simulink model "Non_WindFarm"  (R2024a)
settings: Solver=ode45  StartTime=parSimulacio.ti  StopTime=200  MaxStep=parSimulacio.pas  RelTol=1e-6  AbsTol=1e-6  EnableMultiTasking=on
model workspace (MAT data in the model file):
  tt_vw : Simulink.Parameter (value not decoded)
values from neighbouring files (symbols this model uses):
  L = L'    [Lin_SignalGenerator.m]    (also in Non_ParameterInitialize.m; cal_QR.m = zeros(v, 1); parameters_windFarm2.m)
  nu = size(S, 1)    [Lin_SignalGenerator.m]    (also in Non_ParameterInitialize.m; parameters_windFarm2.m)
  S = zeros(v, v)    [cal_QR.m]
  w0 = [1 -0.00962521549583 0.0254779042049 -0.0160197396127 -0.0156056332727 0.0112137208272 0.0440607583301 -0.0193704893312 -0.0229464276306 -0.00247675309015 0.0285830611299]    [w0.mat]
undefined symbols (not defined in the file or in its folder): parControl, parConvertidor, parGenerador, parGrid, parMecanica, parSimulacio, windspeed
(part 26 of 40)

== system Non_WindFarm/FOM/Wind Farm/Wind Turbine Strings/String6/WT2/WFG/Maquina Sincrona ==
  note: Eq 4.22
  note: park transformation & Inverse
  note: theta_r
  note: Electrical angle=Mechnical angle *Pole Pairs
  note: Omega_r=Omega_m*P
  vsabc : Inport
  omega_m : Inport  Port=2
  theta_m : Inport  Port=3  PortDimensions=1
  Add : Sum  Inputs=+++
  Constant : Constant  Value=-rs/Lq
  Constant1 : Constant  Value=-rs/Ld
  Constant2 : Constant  Value=[1/Lq;0]
  Constant3 : Constant  Value=[1/Lq,0;0,1/Ld]
  Demux : Demux  Outputs=2
  Gain : Gain  Gain=-Ld/Lq
  Gain1 : Gain  Gain=Lq/Ld
  Gain2 : Gain  Gain=-lambda_m
  Gain3 : Gain  Gain=lambda_m
  Gain4 : Gain  Gain=Ld-Lq
  Gain5 : Gain  Gain=3/2*P
  Gain6 : Gain  Gain=P
  Gain7 : Gain  Gain=P
  Integrator : Integrator  InitialCondition=isqd0
  Matrix Concatenate : Concatenate  Mode=Multidimensional array  ConcatenateDimension=2
  Mux : Mux  Inputs=2
  Mux1 : Mux  Inputs=2
  Park : Subsystem
  Product{,2,4..5} (4 alike) : Product  Multiplication=Matrix(*)  RndMeth=Zero
  Product1 : Product  RndMeth=Zero
  Product3 : Product  RndMeth=Zero
  Sum : Sum  Inputs=|++
  isabc : Outport
  parell_m : Outport  Port=2
  wires:
  Constant/1 -> Mux/1
  Gain1/1 -> Mux/2
  Gain/1 -> Mux1/1
  Constant1/1 -> Mux1/2
  omega_m/1 -> Gain6/1
  Mux/1 -> Matrix Concatenate/1
  Mux1/1 -> Matrix Concatenate/2
  Matrix Concatenate/1 -> Product/1
  Product/1 -> Add/1
  Add/1 -> Integrator/1  "disqd"
  Integrator/1 -> Demux/1, Product5/2, Product/2  "isqd"
  Gain2/1 -> Product1/2
  Constant2/1 -> Product1/1
  Product1/1 -> Add/2
  Constant3/1 -> Product2/1
  Product2/1 -> Add/3
  Demux/1 -> Gain3/1, Product3/2
  Product3/1 -> Gain4/1
  Demux/2 -> Product3/1
  Gain3/1 -> Sum/1
  Gain4/1 -> Sum/2
  Sum/1 -> Gain5/1
  Gain5/1 -> parell_m/1
  Gain6/1 -> Gain1/1, Gain/1, Gain2/1
  theta_m/1 -> Gain7/1
  Product4/1 -> Product2/2
  Park/1(Tthetar) -> Product4/1
  Gain7/1 -> Park/1(theta_r)
  Park/2(nTthetar) -> Product5/1
  Product5/1 -> isabc/1
  vsabc/1 -> Product4/2

== system Non_WindFarm/FOM/Wind Farm/Wind Turbine Strings/String6/WT2/WFG/Mecanica nolineal i vent ==
  note: gearbox ration
  note: Gamma_t
  parell_m : Inport
  theta_a : Inport  Port=2
  vw : Inport  Port=3
  Gain1 : Gain  Gain=1/It
  Gain2 : Gain  Gain=nu
  Gain4 : Gain  Gain=nu
  Gain5 : Gain  Gain=nu
  Integrator : Integrator  InitialCondition=omegat0
  Integrator1 : Integrator
  Saturation : Saturate  UpperLimit=inf  LowerLimit=1e-6
  Sum : Sum  Inputs=++|
  Transfer Fcn : TransferFcn  Denominator=[taupitch 1]
  Turbina : Subsystem  mask{rho=1.225, R=R, cs=[0.5 116 0.4 0 0 5 21 0.08 0.035]}
      mask prompts: rho "Densitat de l'aire (Kg/m^3)"; R "Radi (R)"; cs "Constants [c1 c2 .. c9]"
      mask init:
      | A=pi*R^2;
      | c1=cs(1);
      | c2=cs(2);
      | c3=cs(3);
      | c4=cs(4);
      | c5=cs(5);
      | c6=cs(6);
      | c7=cs(7);
      | c8=cs(8);
      | c9=cs(9);
  omega_m : Outport
  theta_m : Outport  Port=2
  Cp : Outport  Port=3
  theta_aleps : Outport  Port=4
  wires:
  Sum/1 -> Gain1/1
  Gain1/1 -> Integrator/1
  Integrator/1 -> Integrator1/1, Gain4/1, Saturation/1
  Turbina/1(parell_turbina) -> Sum/2
  Gain2/1 -> Sum/1
  parell_m/1 -> Gain2/1
  Integrator1/1 -> Gain5/1
  Gain4/1 -> omega_m/1
  Gain5/1 -> theta_m/1
  Saturation/1 -> Turbina/2(omega_aleps)
  Turbina/2(Cp) -> Cp/1
  Transfer Fcn/1 -> theta_aleps/1, Turbina/3(theta_aleps)  "theta_aleps"
  theta_a/1 -> Transfer Fcn/1
  vw/1 -> Turbina/1(velocitat_vent)

== system Non_WindFarm/FOM/Wind Farm/Wind Turbine Strings/String6/WT2/WFG/Park ==
  theta_r : Inport
  Constant4 : Constant  Value=2*pi/3
  Gain7 : Gain  Gain=2/3
  Matrix Concatenate1 : Concatenate  NumInputs=3  Mode=Multidimensional array  ConcatenateDimension=2
  Matrix Concatenate2 : Concatenate  Mode=Multidimensional array  ConcatenateDimension=2
  Mux2 : Mux  Inputs=2
  Mux3 : Mux  Inputs=2
  Mux4 : Mux  Inputs=2
  Mux5 : Mux  Inputs=3
  Mux6 : Mux  Inputs=3
  Sum1 : Sum  Inputs=|++
  Sum2 : Sum  Inputs=|+-
  Trigonometric Function : Trigonometry  Operator=cos
  Trigonometric Function1 : Trigonometry
  Trigonometric Function2 : Trigonometry  Operator=cos
  Trigonometric Function3 : Trigonometry
  Trigonometric Function4 : Trigonometry  Operator=cos
  Trigonometric Function5 : Trigonometry
  Tthetar : Outport
  nTthetar : Outport  Port=2
  wires:
  theta_r/1 -> Sum1/1, Sum2/1, Trigonometric Function/1, Trigonometric Function1/1
  Sum2/1 -> Trigonometric Function2/1, Trigonometric Function3/1
  Sum1/1 -> Trigonometric Function4/1, Trigonometric Function5/1
  Constant4/1 -> Sum2/2, Sum1/2
  Trigonometric Function/1 -> Mux2/1, Mux5/1
  Trigonometric Function1/1 -> Mux2/2, Mux6/1
  Trigonometric Function2/1 -> Mux3/1, Mux5/2
  Trigonometric Function3/1 -> Mux3/2, Mux6/2
  Trigonometric Function4/1 -> Mux4/1, Mux5/3
  Trigonometric Function5/1 -> Mux4/2, Mux6/3
  Mux2/1 -> Matrix Concatenate1/1
  Mux3/1 -> Matrix Concatenate1/2
  Mux4/1 -> Matrix Concatenate1/3
  Matrix Concatenate1/1 -> Gain7/1
  Mux5/1 -> Matrix Concatenate2/1
  Mux6/1 -> Matrix Concatenate2/2
  Gain7/1 -> Tthetar/1
  Matrix Concatenate2/1 -> nTthetar/1

== system Non_WindFarm/FOM/Wind Farm/Wind Turbine Strings/String6/WT3/Transformer-complex/homopolar sequence ==
  note: Vc_cable_abc_bar
  note: Vc_cable_qd_bar
  note: WE
  note: Vc_filter_abc_bar
  note: Vc_filter_qd_bar
  Vc_cable_qd : Inport
  Vc_filter_qd : Inport  Port=2
  Clock : Clock
  Park : Subsystem
  Product{3..5,7} (4 alike) : Product  Multiplication=Matrix(*)  RndMeth=Zero
  homopolar sequence 1 : Subsystem
  homopolar sequence 2 : Subsystem
  we : Gain  Gain=100*pi
  Vc_cable_bar : Outport
  Vc_filter_bar : Outport  Port=2
  wires:
  Park/2(nTthetar) -> Product3/1, Product4/1
  Park/1(Tthetar) -> Product5/1, Product7/1
  Product4/1 -> homopolar sequence 2/1(v)
  homopolar sequence 2/1(v_bar) -> Product7/2
  homopolar sequence 1/1(v_bar) -> Product5/2
  Clock/1 -> we/1
  we/1 -> Park/1(theta_r)
  Product5/1 -> Vc_filter_bar/1
  Vc_cable_qd/1 -> Product4/2
  Vc_filter_qd/1 -> Product3/2
  Product3/1 -> homopolar sequence 1/1(v)
  Product7/1 -> Vc_cable_bar/1

== system Non_WindFarm/FOM/Wind Farm/Wind Turbine Strings/String6/WT3/WFG/Bus Continua1 ==
  note: E=-V_DC?
  note: V_DC/R_DC ?
  note: Eq 5.2-5.5
  ilabc : Inport
  vlabc : Inport  Port=2
  vsabc : Inport  Port=3
  isabc : Inport  Port=4
  Add : Sum  Inputs=+++
  Add1 : Sum  Inputs=+++
  Demux : Demux  Outputs=3
  Demux1 : Demux  Outputs=3
  Divide : Product  Inputs=*/
  Divide1 : Product  Inputs=*/
  Gain : Gain  Gain=1/C
  Integrator : Integrator  InitialCondition=E0  LowerSaturationLimit=10
  Product : Product  RndMeth=Zero
  Product1 : Product  RndMeth=Zero
  Saturation : Saturate  UpperLimit=inf  LowerLimit=1e-3
  Sum : Sum  Inputs=|+-
  E : Outport
  iDCm : Outport  Port=2
  wires:
  Divide1/1 -> Sum/1
  Add1/1 -> Divide1/1
  vlabc/1 -> Product1/2
  Demux1/1 -> Add1/1
  Demux1/2 -> Add1/2
  Product1/1 -> Demux1/1
  ilabc/1 -> Product1/1
  Demux1/3 -> Add1/3
  Integrator/1 -> E/1, Saturation/1
  Saturation/1 -> Divide1/2, Divide/2
  Divide/1 -> Sum/2, iDCm/1
  Add/1 -> Divide/1
  isabc/1 -> Product/2
  vsabc/1 -> Product/1
  Gain/1 -> Integrator/1
  Sum/1 -> Gain/1
  Demux/3 -> Add/3
  Demux/2 -> Add/2
  Demux/1 -> Add/1
  Product/1 -> Demux/1

== system Non_WindFarm/FOM/Wind Farm/Wind Turbine Strings/String6/WT3/WFG/Control Electric Generador ==
  note: voltage source converter
  note: Vs_qd_hat(control output)
  note: 10.14
  note: Vs_qd
  note: 4.25
  note: continuous PI
  note: 4.22
  note: 4.22
  parell_ma : Inport
  Q_sa : Inport  Port=2
  isabc : Inport  Port=3
  omega_m : Inport  Port=4
  theta_m : Inport  Port=5
  Constant1 : Constant  Value=0
  Constant2 : Constant  Value=0
  Constant5 : Constant  Value=0
  Divide : Product  Inputs=*/
  Gain : Gain  Gain=-Lq
  Gain1 : Gain  Gain=Ld
  Gain2 : Gain  Gain=lambda_m
  Gain3 : Gain  Gain=P
  Gain4 : Gain  Gain=2/(3*P)
  Gain5 : Gain  Gain=1/lambda_m
  Gain6 : Gain  Gain=2/3
  Gain7 : Gain  Gain=P
  Gain8 : Gain  Gain=1/lambda_m
  Matrix Concatenate : Concatenate  Mode=Multidimensional array  ConcatenateDimension=2
  Memory : Memory  Commented=through
  Mux{,1..3} (4 alike) : Mux  Inputs=2
  PI : Subsystem
  Park : Subsystem
  Product1 : Product  Multiplication=Matrix(*)  RndMeth=Zero
  Product2 : Product  Multiplication=Matrix(*)  RndMeth=Zero
  Product4 : Product  Multiplication=Matrix(*)  RndMeth=Zero
  Sat inf : Subsystem
  Sum : Sum  Inputs=|++
  Sum1 : Sum  Inputs=|+-
  Sum2 : Sum  Inputs=++|
  vscabc : Outport
  wires:
  Gain7/1 -> Park/1(theta_r)
  Park/1(Tthetar) -> Product4/1
  Constant2/1 -> Mux/1
  Gain1/1 -> Mux/2
  Gain/1 -> Mux1/1
  Constant1/1 -> Mux1/2
  Mux/1 -> Matrix Concatenate/1
  Mux1/1 -> Matrix Concatenate/2
  Matrix Concatenate/1 -> Product1/1
  Product4/1 -> Product1/2, Sum1/2
  omega_m/1 -> Gain3/1
  Product1/1 -> Sum/2
  Sum2/1 -> Product2/2
  Sum1/1 -> PI/1(e)
  PI/1(u) -> Sum2/2
  Mux2/1 -> Sum1/1
  theta_m/1 -> Gain7/1
  isabc/1 -> Product4/2
  Product2/1 -> Memory/1
  Gain3/1 -> Gain1/1, Gain2/1, Gain/1, Sat inf/1(in)
  Mux3/1 -> Sum/1
  Gain2/1 -> Mux3/1
  Constant5/1 -> Mux3/2
  Park/2(nTthetar) -> Product2/1
  Sum/1 -> Sum2/1
  Gain4/1 -> Mux2/1
  Gain5/1 -> Gain4/1
  Gain8/1 -> Gain6/1
  Q_sa/1 -> Divide/1
  Memory/1 -> vscabc/1
  parell_ma/1 -> Gain5/1
  Sat inf/1(out) -> Divide/2
  Divide/1 -> Gain8/1
  Gain6/1 -> Mux2/2

== system Non_WindFarm/FOM/Wind Farm/Wind Turbine Strings/String6/WT3/WFG/Control Electric Tensio ==
  note: 6.12
  note: i_control
  note: Kp Ki, + or - ?
  note: 6.15-6.18
  E : Inport
  IDCm : Inport  Port=2
  E* : Constant  Value=Easterisc
  Sum : Sum  Inputs=|++
  Sum1 : Sum  Inputs=|+-
  Transfer Fcn : TransferFcn  Numerator=[Kp Ki]  Denominator=[1 0]
  iDCla : Outport
  wires:
  IDCm/1 -> Sum/2
  Sum1/1 -> Transfer Fcn/1
  E/1 -> Sum1/2
  Sum/1 -> iDCla/1
  Transfer Fcn/1 -> Sum/1
  E*/1 -> Sum1/1

== system Non_WindFarm/FOM/Wind Farm/Wind Turbine Strings/String6/WT3/WFG/Control Mecanic ==
  note: Eq 2.19 ???
  note: ??? theta_a?
  note: Generator nominal speed Wmn
  omega_m : Inport
  Constant : Constant  Value=omegamn
  Gain : Gain  Gain=-KCP
  Math Function : Math  Operator=square  SignedPower=on
  Saturation : Saturate  UpperLimit=inf  LowerLimit=0
  Saturation1 : Saturate  UpperLimit=90  LowerLimit=0
  Subtract : Sum  Inputs=+-
  Transfer Fcn : TransferFcn  Numerator=[Kp Ki]  Denominator=[1 0]
  parell_ma : Outport
  theta_a : Outport  Port=2
  wires:
  omega_m/1 -> Subtract/1, Math Function/1
  Math Function/1 -> Gain/1
  Gain/1 -> parell_ma/1
  Saturation1/1 -> theta_a/1
  Constant/1 -> Subtract/2
  Subtract/1 -> Saturation/1
  Saturation/1 -> Transfer Fcn/1
  Transfer Fcn/1 -> Saturation1/1

== system Non_WindFarm/FOM/Wind Farm/Wind Turbine Strings/String6/WT3/WFG/Control de Corrent de Xarxa2 ==
  vzabc : Inport
  ilabc : Inport  Port=2
  iDCla : Inport  Port=3
  E : Inport  Port=4
  Constant1 : Constant  Value=2*pi*50
  Constant2 : Constant  Value=0
  Constant3 : Constant  Value=[2,-1,-1;0,-sqrt(3),sqrt(3)]
  Constant5 : Constant  Value=2*pi*50
  Constant6 : Constant  Value=[0;0]
  Demux : Demux  Outputs=2
  Demux1 : Demux  Outputs=2
  Divide : Product  Inputs=*/
  Gain1 : Gain  Gain=2/3
  Gain12 : Gain
  Gain2 : Gain  Gain=Ll
  Gain4 : Gain  Gain=Ll
  Gain6 : Gain  Gain=1/3
  Integrator : Integrator
  Memory : Memory  Commented=through
  Mux : Mux  Inputs=2
  Mux1 : Mux  Inputs=2
  PI_d : Subsystem
  Product : Product  RndMeth=Zero
  Product{1..2,11..13} (5 alike) : Product  Multiplication=Matrix(*)  RndMeth=Zero
  Product10 : Product  RndMeth=Zero
  Product3 : Product  RndMeth=Zero
  Scope : Scope
  Selector : Selector  InputPortWidth=2  IndexOptions=Index vector (dialog)  Indices=[1]  OutputSizes=1
  Selector2 : Selector  InputPortWidth=2  IndexOptions=Index vector (dialog)  Indices=[2]  OutputSizes=1
  Step : Step  Time=1e-3  Before=1  After=0  SampleTime=0
  Sum1 : Sum  Inputs=-+|
  Sum2 : Sum  Inputs=+--
  Sum3 : Sum  Inputs=+-
  Sum9 : Sum  Inputs=++|
  Switch : Switch  Criteria=u2 > Threshold  SaturateOnIntegerOverflow=off  InputSameDT=off
  Transfer Fcn : TransferFcn  Numerator=-[1 0.129]  Denominator=[1 0]
  rotacio1 : Subsystem
  vlabc : Outport
  wires:
  Integrator/1 -> rotacio1/1(theta)
  E/1 -> Product10/1
  iDCla/1 -> Product10/2
  PI_d/1(u) -> Demux/1
  Demux/1 -> Sum2/3
  Demux/2 -> Sum3/2
  Sum3/1 -> Mux1/2
  Sum2/1 -> Mux1/1
  Product/1 -> Gain2/1
  Product3/1 -> Gain4/1
  Demux1/2 -> Product3/2
  Demux1/1 -> Product/2
  Gain1/1 -> Mux/1
  Gain4/1 -> Sum2/2
  Gain2/1 -> Sum3/1
  Constant2/1 -> Mux/2
  Memory/1 -> vlabc/1
  Constant1/1 -> Product/1, Product3/1
  Product11/1 -> Product1/2
  Product1/1 -> Scope/1, Selector/1, Selector2/1
  Mux/1 -> Sum1/2
  Product13/1 -> Demux1/1, Sum1/1
  Selector/1 -> Divide/2, Sum2/1
  Mux1/1 -> Product2/2
  rotacio1/2(nT) -> Product2/1
  Divide/1 -> Gain1/1
  Product10/1 -> Divide/1
  Product2/1 -> Memory/1
  Switch/1 -> PI_d/1(e)
  Sum1/1 -> Switch/3
  Constant6/1 -> Switch/1
  Step/1 -> Gain12/1
  Gain12/1 -> Switch/2
  Sum9/1 -> Integrator/1
  Selector2/1 -> Transfer Fcn/1
  Constant5/1 -> Sum9/1
  Transfer Fcn/1 -> Sum9/2
  Constant3/1 -> Gain6/1
  Gain6/1 -> Product12/1, Product11/1
  vzabc/1 -> Product11/2
  ilabc/1 -> Product12/2
  Product12/1 -> Product13/2
  rotacio1/1(T) -> Product13/1, Product1/1

== system Non_WindFarm/FOM/Wind Farm/Wind Turbine Strings/String6/WT3/WFG/Filtre de Xarxa1 ==
  note: Vnl and Vnz? Eq 5.11
  vzabc : Inport
  vlabc : Inport  Port=2
  Gain2 : Gain  Gain=rl
  Gain3 : Gain  Gain=1/Ll
  Integrator : Integrator  InitialCondition=[0;0;0]
  Sum : Sum  Inputs=|+-
  Sum1 : Sum  Inputs=|+-
  ilabc : Outport
  wires:
  vlabc/1 -> Sum/2
  vzabc/1 -> Sum/1
  Gain3/1 -> Integrator/1
  Integrator/1 -> ilabc/1, Gain2/1
  Sum1/1 -> Gain3/1
  Gain2/1 -> Sum1/2
  Sum/1 -> Sum1/1

== system Non_WindFarm/FOM/Wind Farm/Wind Turbine Strings/String6/WT3/WFG/Maquina Sincrona ==
  note: Eq 4.22
  note: park transformation & Inverse
  note: theta_r
  note: Electrical angle=Mechnical angle *Pole Pairs
  note: Omega_r=Omega_m*P
  vsabc : Inport
  omega_m : Inport  Port=2
  theta_m : Inport  Port=3  PortDimensions=1
  Add : Sum  Inputs=+++
  Constant : Constant  Value=-rs/Lq
  Constant1 : Constant  Value=-rs/Ld
  Constant2 : Constant  Value=[1/Lq;0]
  Constant3 : Constant  Value=[1/Lq,0;0,1/Ld]
  Demux : Demux  Outputs=2
  Gain : Gain  Gain=-Ld/Lq
  Gain1 : Gain  Gain=Lq/Ld
  Gain2 : Gain  Gain=-lambda_m
  Gain3 : Gain  Gain=lambda_m
  Gain4 : Gain  Gain=Ld-Lq
  Gain5 : Gain  Gain=3/2*P
  Gain6 : Gain  Gain=P
  Gain7 : Gain  Gain=P
  Integrator : Integrator  InitialCondition=isqd0
  Matrix Concatenate : Concatenate  Mode=Multidimensional array  ConcatenateDimension=2
  Mux : Mux  Inputs=2
  Mux1 : Mux  Inputs=2
  Park : Subsystem
  Product{,2,4..5} (4 alike) : Product  Multiplication=Matrix(*)  RndMeth=Zero
  Product1 : Product  RndMeth=Zero
  Product3 : Product  RndMeth=Zero
  Sum : Sum  Inputs=|++
  isabc : Outport
  parell_m : Outport  Port=2
  wires:
  Constant/1 -> Mux/1
  Gain1/1 -> Mux/2
  Gain/1 -> Mux1/1
  Constant1/1 -> Mux1/2
  omega_m/1 -> Gain6/1
  Mux/1 -> Matrix Concatenate/1
  Mux1/1 -> Matrix Concatenate/2
  Matrix Concatenate/1 -> Product/1
  Product/1 -> Add/1
  Add/1 -> Integrator/1  "disqd"
  Integrator/1 -> Demux/1, Product5/2, Product/2  "isqd"
  Gain2/1 -> Product1/2
  Constant2/1 -> Product1/1
  Product1/1 -> Add/2
  Constant3/1 -> Product2/1
  Product2/1 -> Add/3
  Demux/1 -> Gain3/1, Product3/2
  Product3/1 -> Gain4/1
  Demux/2 -> Product3/1
  Gain3/1 -> Sum/1
  Gain4/1 -> Sum/2
  Sum/1 -> Gain5/1
  Gain5/1 -> parell_m/1
  Gain6/1 -> Gain1/1, Gain/1, Gain2/1
  theta_m/1 -> Gain7/1
  Product4/1 -> Product2/2
  Park/1(Tthetar) -> Product4/1
  Gain7/1 -> Park/1(theta_r)
  Park/2(nTthetar) -> Product5/1
  Product5/1 -> isabc/1
  vsabc/1 -> Product4/2

== system Non_WindFarm/FOM/Wind Farm/Wind Turbine Strings/String6/WT3/WFG/Mecanica nolineal i vent ==
  note: gearbox ration
  note: Gamma_t
  parell_m : Inport
  theta_a : Inport  Port=2
  vw : Inport  Port=3
  Gain1 : Gain  Gain=1/It
  Gain2 : Gain  Gain=nu
  Gain4 : Gain  Gain=nu
  Gain5 : Gain  Gain=nu
  Integrator : Integrator  InitialCondition=omegat0
  Integrator1 : Integrator
  Saturation : Saturate  UpperLimit=inf  LowerLimit=1e-6
  Sum : Sum  Inputs=++|
  Transfer Fcn : TransferFcn  Denominator=[taupitch 1]
  Turbina : Subsystem  mask{rho=1.225, R=R, cs=[0.5 116 0.4 0 0 5 21 0.08 0.035]}
      mask prompts: rho "Densitat de l'aire (Kg/m^3)"; R "Radi (R)"; cs "Constants [c1 c2 .. c9]"
      mask init:
      | A=pi*R^2;
      | c1=cs(1);
      | c2=cs(2);
      | c3=cs(3);
      | c4=cs(4);
      | c5=cs(5);
      | c6=cs(6);
      | c7=cs(7);
      | c8=cs(8);
      | c9=cs(9);
  omega_m : Outport
  theta_m : Outport  Port=2
  Cp : Outport  Port=3
  theta_aleps : Outport  Port=4
  wires:
  Sum/1 -> Gain1/1
  Gain1/1 -> Integrator/1
  Integrator/1 -> Integrator1/1, Gain4/1, Saturation/1
  Turbina/1(parell_turbina) -> Sum/2
  Gain2/1 -> Sum/1
  parell_m/1 -> Gain2/1
  Integrator1/1 -> Gain5/1
  Gain4/1 -> omega_m/1
  Gain5/1 -> theta_m/1
  Saturation/1 -> Turbina/2(omega_aleps)
  Turbina/2(Cp) -> Cp/1
  Transfer Fcn/1 -> theta_aleps/1, Turbina/3(theta_aleps)  "theta_aleps"
  theta_a/1 -> Transfer Fcn/1
  vw/1 -> Turbina/1(velocitat_vent)

== system Non_WindFarm/FOM/Wind Farm/Wind Turbine Strings/String6/WT3/WFG/Park ==
  theta_r : Inport
  Constant4 : Constant  Value=2*pi/3
  Gain7 : Gain  Gain=2/3
  Matrix Concatenate1 : Concatenate  NumInputs=3  Mode=Multidimensional array  ConcatenateDimension=2
  Matrix Concatenate2 : Concatenate  Mode=Multidimensional array  ConcatenateDimension=2
  Mux2 : Mux  Inputs=2
  Mux3 : Mux  Inputs=2
  Mux4 : Mux  Inputs=2
  Mux5 : Mux  Inputs=3
  Mux6 : Mux  Inputs=3
  Sum1 : Sum  Inputs=|++
  Sum2 : Sum  Inputs=|+-
  Trigonometric Function : Trigonometry  Operator=cos
  Trigonometric Function1 : Trigonometry
  Trigonometric Function2 : Trigonometry  Operator=cos
  Trigonometric Function3 : Trigonometry
  Trigonometric Function4 : Trigonometry  Operator=cos
  Trigonometric Function5 : Trigonometry
  Tthetar : Outport
  nTthetar : Outport  Port=2
  wires:
  theta_r/1 -> Sum1/1, Sum2/1, Trigonometric Function/1, Trigonometric Function1/1
  Sum2/1 -> Trigonometric Function2/1, Trigonometric Function3/1
  Sum1/1 -> Trigonometric Function4/1, Trigonometric Function5/1
  Constant4/1 -> Sum2/2, Sum1/2
  Trigonometric Function/1 -> Mux2/1, Mux5/1
  Trigonometric Function1/1 -> Mux2/2, Mux6/1
  Trigonometric Function2/1 -> Mux3/1, Mux5/2
  Trigonometric Function3/1 -> Mux3/2, Mux6/2
  Trigonometric Function4/1 -> Mux4/1, Mux5/3
  Trigonometric Function5/1 -> Mux4/2, Mux6/3
  Mux2/1 -> Matrix Concatenate1/1
  Mux3/1 -> Matrix Concatenate1/2
  Mux4/1 -> Matrix Concatenate1/3
  Matrix Concatenate1/1 -> Gain7/1
  Mux5/1 -> Matrix Concatenate2/1
  Mux6/1 -> Matrix Concatenate2/2
  Gain7/1 -> Tthetar/1
  Matrix Concatenate2/1 -> nTthetar/1

== system Non_WindFarm/FOM/Wind Farm/Wind Turbine Strings/String6/WT4/Transformer-complex/homopolar sequence ==
  note: Vc_filter_qd_bar
  note: Vc_filter_abc_bar
  note: WE
  note: Vc_cable_qd_bar
  note: Vc_cable_abc_bar
  Vc_cable_qd : Inport
  Vc_filter_qd : Inport  Port=2
  Clock : Clock
  Park : Subsystem
  Product{3..5,7} (4 alike) : Product  Multiplication=Matrix(*)  RndMeth=Zero
  homopolar sequence 1 : Subsystem
  homopolar sequence 2 : Subsystem
  we : Gain  Gain=100*pi
  Vc_cable_bar : Outport
  Vc_filter_bar : Outport  Port=2
  wires:
  Product7/1 -> Vc_cable_bar/1
  Product3/1 -> homopolar sequence 1/1(v)
  Vc_filter_qd/1 -> Product3/2
  Vc_cable_qd/1 -> Product4/2
  Product5/1 -> Vc_filter_bar/1
  we/1 -> Park/1(theta_r)
  Clock/1 -> we/1
  homopolar sequence 1/1(v_bar) -> Product5/2
  homopolar sequence 2/1(v_bar) -> Product7/2
  Product4/1 -> homopolar sequence 2/1(v)
  Park/1(Tthetar) -> Product7/1, Product5/1
  Park/2(nTthetar) -> Product4/1, Product3/1

== system Non_WindFarm/FOM/Wind Farm/Wind Turbine Strings/String6/WT4/WFG/Bus Continua1 ==
  note: E=-V_DC?
  note: V_DC/R_DC ?
  note: Eq 5.2-5.5
  ilabc : Inport
  vlabc : Inport  Port=2
  vsabc : Inport  Port=3
  isabc : Inport  Port=4
  Add : Sum  Inputs=+++
  Add1 : Sum  Inputs=+++
  Demux : Demux  Outputs=3
  Demux1 : Demux  Outputs=3
  Divide : Product  Inputs=*/
  Divide1 : Product  Inputs=*/
  Gain : Gain  Gain=1/C
  Integrator : Integrator  InitialCondition=E0  LowerSaturationLimit=10
  Product : Product  RndMeth=Zero
  Product1 : Product  RndMeth=Zero
  Saturation : Saturate  UpperLimit=inf  LowerLimit=1e-3
  Sum : Sum  Inputs=|+-
  E : Outport
  iDCm : Outport  Port=2
  wires:
  Divide1/1 -> Sum/1
  Add1/1 -> Divide1/1
  vlabc/1 -> Product1/2
  Demux1/1 -> Add1/1
  Demux1/2 -> Add1/2
  Product1/1 -> Demux1/1
  ilabc/1 -> Product1/1
  Demux1/3 -> Add1/3
  Integrator/1 -> E/1, Saturation/1
  Saturation/1 -> Divide1/2, Divide/2
  Divide/1 -> Sum/2, iDCm/1
  Add/1 -> Divide/1
  isabc/1 -> Product/2
  vsabc/1 -> Product/1
  Gain/1 -> Integrator/1
  Sum/1 -> Gain/1
  Demux/3 -> Add/3
  Demux/2 -> Add/2
  Demux/1 -> Add/1
  Product/1 -> Demux/1

== system Non_WindFarm/FOM/Wind Farm/Wind Turbine Strings/String6/WT4/WFG/Control Electric Generador ==
  note: voltage source converter
  note: Vs_qd_hat(control output)
  note: 10.14
  note: Vs_qd
  note: 4.25
  note: continuous PI
  note: 4.22
  note: 4.22
  parell_ma : Inport
  Q_sa : Inport  Port=2
  isabc : Inport  Port=3
  omega_m : Inport  Port=4
  theta_m : Inport  Port=5
  Constant1 : Constant  Value=0
  Constant2 : Constant  Value=0
  Constant5 : Constant  Value=0
  Divide : Product  Inputs=*/
  Gain : Gain  Gain=-Lq
  Gain1 : Gain  Gain=Ld
  Gain2 : Gain  Gain=lambda_m
  Gain3 : Gain  Gain=P
  Gain4 : Gain  Gain=2/(3*P)
  Gain5 : Gain  Gain=1/lambda_m
  Gain6 : Gain  Gain=2/3
  Gain7 : Gain  Gain=P
  Gain8 : Gain  Gain=1/lambda_m
  Matrix Concatenate : Concatenate  Mode=Multidimensional array  ConcatenateDimension=2
  Memory : Memory  Commented=through
  Mux{,1..3} (4 alike) : Mux  Inputs=2
  PI : Subsystem
  Park : Subsystem
  Product1 : Product  Multiplication=Matrix(*)  RndMeth=Zero
  Product2 : Product  Multiplication=Matrix(*)  RndMeth=Zero
  Product4 : Product  Multiplication=Matrix(*)  RndMeth=Zero
  Sat inf : Subsystem
  Sum : Sum  Inputs=|++
  Sum1 : Sum  Inputs=|+-
  Sum2 : Sum  Inputs=++|
  vscabc : Outport
  wires:
  Gain7/1 -> Park/1(theta_r)
  Park/1(Tthetar) -> Product4/1
  Constant2/1 -> Mux/1
  Gain1/1 -> Mux/2
  Gain/1 -> Mux1/1
  Constant1/1 -> Mux1/2
  Mux/1 -> Matrix Concatenate/1
  Mux1/1 -> Matrix Concatenate/2
  Matrix Concatenate/1 -> Product1/1
  Product4/1 -> Product1/2, Sum1/2
  omega_m/1 -> Gain3/1
  Product1/1 -> Sum/2
  Sum2/1 -> Product2/2
  Sum1/1 -> PI/1(e)
  PI/1(u) -> Sum2/2
  Mux2/1 -> Sum1/1
  theta_m/1 -> Gain7/1
  isabc/1 -> Product4/2
  Product2/1 -> Memory/1
  Gain3/1 -> Gain1/1, Gain2/1, Gain/1, Sat inf/1(in)
  Mux3/1 -> Sum/1
  Gain2/1 -> Mux3/1
  Constant5/1 -> Mux3/2
  Park/2(nTthetar) -> Product2/1
  Sum/1 -> Sum2/1
  Gain4/1 -> Mux2/1
  Gain5/1 -> Gain4/1
  Gain8/1 -> Gain6/1
  Q_sa/1 -> Divide/1
  Memory/1 -> vscabc/1
  parell_ma/1 -> Gain5/1
  Sat inf/1(out) -> Divide/2
  Divide/1 -> Gain8/1
  Gain6/1 -> Mux2/2

== system Non_WindFarm/FOM/Wind Farm/Wind Turbine Strings/String6/WT4/WFG/Control Electric Tensio ==
  note: 6.12
  note: i_control
  note: Kp Ki, + or - ?
  note: 6.15-6.18
  E : Inport
  IDCm : Inport  Port=2
  E* : Constant  Value=Easterisc
  Sum : Sum  Inputs=|++
  Sum1 : Sum  Inputs=|+-
  Transfer Fcn : TransferFcn  Numerator=[Kp Ki]  Denominator=[1 0]
  iDCla : Outport
  wires:
  IDCm/1 -> Sum/2
  Sum1/1 -> Transfer Fcn/1
  E/1 -> Sum1/2
  Sum/1 -> iDCla/1
  Transfer Fcn/1 -> Sum/1
  E*/1 -> Sum1/1

== system Non_WindFarm/FOM/Wind Farm/Wind Turbine Strings/String6/WT4/WFG/Control Mecanic ==
  note: Eq 2.19 ???
  note: ??? theta_a?
  note: Generator nominal speed Wmn
  omega_m : Inport
  Constant : Constant  Value=omegamn
  Gain : Gain  Gain=-KCP
  Math Function : Math  Operator=square  SignedPower=on
  Saturation : Saturate  UpperLimit=inf  LowerLimit=0
  Saturation1 : Saturate  UpperLimit=90  LowerLimit=0
  Subtract : Sum  Inputs=+-
  Transfer Fcn : TransferFcn  Numerator=[Kp Ki]  Denominator=[1 0]
  parell_ma : Outport
  theta_a : Outport  Port=2
  wires:
  omega_m/1 -> Subtract/1, Math Function/1
  Math Function/1 -> Gain/1
  Gain/1 -> parell_ma/1
  Saturation1/1 -> theta_a/1
  Constant/1 -> Subtract/2
  Subtract/1 -> Saturation/1
  Saturation/1 -> Transfer Fcn/1
  Transfer Fcn/1 -> Saturation1/1

== system Non_WindFarm/FOM/Wind Farm/Wind Turbine Strings/String6/WT4/WFG/Control de Corrent de Xarxa2 ==
  vzabc : Inport
  ilabc : Inport  Port=2
  iDCla : Inport  Port=3
  E : Inport  Port=4
  Constant1 : Constant  Value=2*pi*50
  Constant2 : Constant  Value=0
  Constant3 : Constant  Value=[2,-1,-1;0,-sqrt(3),sqrt(3)]
  Constant5 : Constant  Value=2*pi*50
  Constant6 : Constant  Value=[0;0]
  Demux : Demux  Outputs=2
  Demux1 : Demux  Outputs=2
  Divide : Product  Inputs=*/
  Gain1 : Gain  Gain=2/3
  Gain12 : Gain
  Gain2 : Gain  Gain=Ll
  Gain4 : Gain  Gain=Ll
  Gain6 : Gain  Gain=1/3
  Integrator : Integrator
  Memory : Memory  Commented=through
  Mux : Mux  Inputs=2
  Mux1 : Mux  Inputs=2
  PI_d : Subsystem
  Product : Product  RndMeth=Zero
  Product{1..2,11..13} (5 alike) : Product  Multiplication=Matrix(*)  RndMeth=Zero
  Product10 : Product  RndMeth=Zero
  Product3 : Product  RndMeth=Zero
  Scope : Scope
  Selector : Selector  InputPortWidth=2  IndexOptions=Index vector (dialog)  Indices=[1]  OutputSizes=1
  Selector2 : Selector  InputPortWidth=2  IndexOptions=Index vector (dialog)  Indices=[2]  OutputSizes=1
  Step : Step  Time=1e-3  Before=1  After=0  SampleTime=0
  Sum1 : Sum  Inputs=-+|
  Sum2 : Sum  Inputs=+--
  Sum3 : Sum  Inputs=+-
  Sum9 : Sum  Inputs=++|
  Switch : Switch  Criteria=u2 > Threshold  SaturateOnIntegerOverflow=off  InputSameDT=off
  Transfer Fcn : TransferFcn  Numerator=-[1 0.129]  Denominator=[1 0]
  rotacio1 : Subsystem
  vlabc : Outport
  wires:
  Integrator/1 -> rotacio1/1(theta)
  E/1 -> Product10/1
  iDCla/1 -> Product10/2
  PI_d/1(u) -> Demux/1
  Demux/1 -> Sum2/3
  Demux/2 -> Sum3/2
  Sum3/1 -> Mux1/2
  Sum2/1 -> Mux1/1
  Product/1 -> Gain2/1
  Product3/1 -> Gain4/1
  Demux1/2 -> Product3/2
  Demux1/1 -> Product/2
  Gain1/1 -> Mux/1
  Gain4/1 -> Sum2/2
  Gain2/1 -> Sum3/1
  Constant2/1 -> Mux/2
  Memory/1 -> vlabc/1
  Constant1/1 -> Product/1, Product3/1
  Product11/1 -> Product1/2
  Product1/1 -> Scope/1, Selector/1, Selector2/1
  Mux/1 -> Sum1/2
  Product13/1 -> Demux1/1, Sum1/1
  Selector/1 -> Divide/2, Sum2/1
  Mux1/1 -> Product2/2
  rotacio1/2(nT) -> Product2/1
  Divide/1 -> Gain1/1
  Product10/1 -> Divide/1
  Product2/1 -> Memory/1
  Switch/1 -> PI_d/1(e)
  Sum1/1 -> Switch/3
  Constant6/1 -> Switch/1
  Step/1 -> Gain12/1
  Gain12/1 -> Switch/2
  Sum9/1 -> Integrator/1
  Selector2/1 -> Transfer Fcn/1
  Constant5/1 -> Sum9/1
  Transfer Fcn/1 -> Sum9/2
  Constant3/1 -> Gain6/1
  Gain6/1 -> Product12/1, Product11/1
  vzabc/1 -> Product11/2
  ilabc/1 -> Product12/2
  Product12/1 -> Product13/2
  rotacio1/1(T) -> Product13/1, Product1/1

== system Non_WindFarm/FOM/Wind Farm/Wind Turbine Strings/String6/WT4/WFG/Filtre de Xarxa1 ==
  note: Vnl and Vnz? Eq 5.11
  vzabc : Inport
  vlabc : Inport  Port=2
  Gain2 : Gain  Gain=rl
  Gain3 : Gain  Gain=1/Ll
  Integrator : Integrator  InitialCondition=[0;0;0]
  Sum : Sum  Inputs=|+-
  Sum1 : Sum  Inputs=|+-
  ilabc : Outport
  wires:
  vlabc/1 -> Sum/2
  vzabc/1 -> Sum/1
  Gain3/1 -> Integrator/1
  Integrator/1 -> ilabc/1, Gain2/1
  Sum1/1 -> Gain3/1
  Gain2/1 -> Sum1/2
  Sum/1 -> Sum1/1

== system Non_WindFarm/FOM/Wind Farm/Wind Turbine Strings/String6/WT4/WFG/Maquina Sincrona ==
  note: Eq 4.22
  note: park transformation & Inverse
  note: theta_r
  note: Electrical angle=Mechnical angle *Pole Pairs
  note: Omega_r=Omega_m*P
  vsabc : Inport
  omega_m : Inport  Port=2
  theta_m : Inport  Port=3  PortDimensions=1
  Add : Sum  Inputs=+++
  Constant : Constant  Value=-rs/Lq
  Constant1 : Constant  Value=-rs/Ld
  Constant2 : Constant  Value=[1/Lq;0]
  Constant3 : Constant  Value=[1/Lq,0;0,1/Ld]
  Demux : Demux  Outputs=2
  Gain : Gain  Gain=-Ld/Lq
  Gain1 : Gain  Gain=Lq/Ld
  Gain2 : Gain  Gain=-lambda_m
  Gain3 : Gain  Gain=lambda_m
  Gain4 : Gain  Gain=Ld-Lq
  Gain5 : Gain  Gain=3/2*P
  Gain6 : Gain  Gain=P
  Gain7 : Gain  Gain=P
  Integrator : Integrator  InitialCondition=isqd0
  Matrix Concatenate : Concatenate  Mode=Multidimensional array  ConcatenateDimension=2
  Mux : Mux  Inputs=2
  Mux1 : Mux  Inputs=2
  Park : Subsystem
  Product{,2,4..5} (4 alike) : Product  Multiplication=Matrix(*)  RndMeth=Zero
  Product1 : Product  RndMeth=Zero
  Product3 : Product  RndMeth=Zero
  Sum : Sum  Inputs=|++
  isabc : Outport
  parell_m : Outport  Port=2
  wires:
  Constant/1 -> Mux/1
  Gain1/1 -> Mux/2
  Gain/1 -> Mux1/1
  Constant1/1 -> Mux1/2
  omega_m/1 -> Gain6/1
  Mux/1 -> Matrix Concatenate/1
  Mux1/1 -> Matrix Concatenate/2
  Matrix Concatenate/1 -> Product/1
  Product/1 -> Add/1
  Add/1 -> Integrator/1  "disqd"
  Integrator/1 -> Demux/1, Product5/2, Product/2  "isqd"
  Gain2/1 -> Product1/2
  Constant2/1 -> Product1/1
  Product1/1 -> Add/2
  Constant3/1 -> Product2/1
  Product2/1 -> Add/3
  Demux/1 -> Gain3/1, Product3/2
  Product3/1 -> Gain4/1
  Demux/2 -> Product3/1
  Gain3/1 -> Sum/1
  Gain4/1 -> Sum/2
  Sum/1 -> Gain5/1
  Gain5/1 -> parell_m/1
  Gain6/1 -> Gain1/1, Gain/1, Gain2/1
  theta_m/1 -> Gain7/1
  Product4/1 -> Product2/2
  Park/1(Tthetar) -> Product4/1
  Gain7/1 -> Park/1(theta_r)
  Park/2(nTthetar) -> Product5/1
  Product5/1 -> isabc/1
  vsabc/1 -> Product4/2

== system Non_WindFarm/FOM/Wind Farm/Wind Turbine Strings/String6/WT4/WFG/Mecanica nolineal i vent ==
  note: gearbox ration
  note: Gamma_t
  parell_m : Inport
  theta_a : Inport  Port=2
  vw : Inport  Port=3
  Gain1 : Gain  Gain=1/It
  Gain2 : Gain  Gain=nu
  Gain4 : Gain  Gain=nu
  Gain5 : Gain  Gain=nu
  Integrator : Integrator  InitialCondition=omegat0
  Integrator1 : Integrator
  Saturation : Saturate  UpperLimit=inf  LowerLimit=1e-6
  Sum : Sum  Inputs=++|
  Transfer Fcn : TransferFcn  Denominator=[taupitch 1]
  Turbina : Subsystem  mask{rho=1.225, R=R, cs=[0.5 116 0.4 0 0 5 21 0.08 0.035]}
      mask prompts: rho "Densitat de l'aire (Kg/m^3)"; R "Radi (R)"; cs "Constants [c1 c2 .. c9]"
      mask init:
      | A=pi*R^2;
      | c1=cs(1);
      | c2=cs(2);
      | c3=cs(3);
      | c4=cs(4);
      | c5=cs(5);
      | c6=cs(6);
      | c7=cs(7);
      | c8=cs(8);
      | c9=cs(9);
  omega_m : Outport
  theta_m : Outport  Port=2
  Cp : Outport  Port=3
  theta_aleps : Outport  Port=4
  wires:
  Sum/1 -> Gain1/1
  Gain1/1 -> Integrator/1
  Integrator/1 -> Integrator1/1, Gain4/1, Saturation/1
  Turbina/1(parell_turbina) -> Sum/2
  Gain2/1 -> Sum/1
  parell_m/1 -> Gain2/1
  Integrator1/1 -> Gain5/1
  Gain4/1 -> omega_m/1
  Gain5/1 -> theta_m/1
  Saturation/1 -> Turbina/2(omega_aleps)
  Turbina/2(Cp) -> Cp/1
  Transfer Fcn/1 -> theta_aleps/1, Turbina/3(theta_aleps)  "theta_aleps"
  theta_a/1 -> Transfer Fcn/1
  vw/1 -> Turbina/1(velocitat_vent)

== system Non_WindFarm/FOM/Wind Farm/Wind Turbine Strings/String6/WT4/WFG/Park ==
  theta_r : Inport
  Constant4 : Constant  Value=2*pi/3
  Gain7 : Gain  Gain=2/3
  Matrix Concatenate1 : Concatenate  NumInputs=3  Mode=Multidimensional array  ConcatenateDimension=2
  Matrix Concatenate2 : Concatenate  Mode=Multidimensional array  ConcatenateDimension=2
  Mux2 : Mux  Inputs=2
  Mux3 : Mux  Inputs=2
  Mux4 : Mux  Inputs=2
  Mux5 : Mux  Inputs=3
  Mux6 : Mux  Inputs=3
  Sum1 : Sum  Inputs=|++
  Sum2 : Sum  Inputs=|+-
  Trigonometric Function : Trigonometry  Operator=cos
  Trigonometric Function1 : Trigonometry
  Trigonometric Function2 : Trigonometry  Operator=cos
  Trigonometric Function3 : Trigonometry
  Trigonometric Function4 : Trigonometry  Operator=cos
  Trigonometric Function5 : Trigonometry
  Tthetar : Outport
  nTthetar : Outport  Port=2
  wires:
  theta_r/1 -> Sum1/1, Sum2/1, Trigonometric Function/1, Trigonometric Function1/1
  Sum2/1 -> Trigonometric Function2/1, Trigonometric Function3/1
  Sum1/1 -> Trigonometric Function4/1, Trigonometric Function5/1
  Constant4/1 -> Sum2/2, Sum1/2
  Trigonometric Function/1 -> Mux2/1, Mux5/1
  Trigonometric Function1/1 -> Mux2/2, Mux6/1
  Trigonometric Function2/1 -> Mux3/1, Mux5/2
  Trigonometric Function3/1 -> Mux3/2, Mux6/2
  Trigonometric Function4/1 -> Mux4/1, Mux5/3
  Trigonometric Function5/1 -> Mux4/2, Mux6/3
  Mux2/1 -> Matrix Concatenate1/1
  Mux3/1 -> Matrix Concatenate1/2
  Mux4/1 -> Matrix Concatenate1/3
  Matrix Concatenate1/1 -> Gain7/1
  Mux5/1 -> Matrix Concatenate2/1
  Mux6/1 -> Matrix Concatenate2/2
  Gain7/1 -> Tthetar/1
  Matrix Concatenate2/1 -> nTthetar/1

== system Non_WindFarm/FOM/Wind Farm/Wind Turbine Strings/String6/WT5/Transformer-complex/homopolar sequence ==
  note: Vc_cable_abc_bar
  note: Vc_cable_qd_bar
  note: WE
  note: Vc_filter_abc_bar
  note: Vc_filter_qd_bar
  Vc_cable_qd : Inport
  Vc_filter_qd : Inport  Port=2
  Clock : Clock
  Park : Subsystem
  Product{3..5,7} (4 alike) : Product  Multiplication=Matrix(*)  RndMeth=Zero
  homopolar sequence 1 : Subsystem
  homopolar sequence 2 : Subsystem
  we : Gain  Gain=100*pi
  Vc_cable_bar : Outport
  Vc_filter_bar : Outport  Port=2
  wires:
  Park/2(nTthetar) -> Product3/1, Product4/1
  Park/1(Tthetar) -> Product5/1, Product7/1
  Product4/1 -> homopolar sequence 2/1(v)
  homopolar sequence 2/1(v_bar) -> Product7/2
  homopolar sequence 1/1(v_bar) -> Product5/2
  Clock/1 -> we/1
  we/1 -> Park/1(theta_r)
  Product5/1 -> Vc_filter_bar/1
  Vc_cable_qd/1 -> Product4/2
  Vc_filter_qd/1 -> Product3/2
  Product3/1 -> homopolar sequence 1/1(v)
  Product7/1 -> Vc_cable_bar/1

== system Non_WindFarm/FOM/Wind Farm/Wind Turbine Strings/String6/WT5/WFG/Bus Continua1 ==
  note: E=-V_DC?
  note: V_DC/R_DC ?
  note: Eq 5.2-5.5
  ilabc : Inport
  vlabc : Inport  Port=2
  vsabc : Inport  Port=3
  isabc : Inport  Port=4
  Add : Sum  Inputs=+++
  Add1 : Sum  Inputs=+++
  Demux : Demux  Outputs=3
  Demux1 : Demux  Outputs=3
  Divide : Product  Inputs=*/
  Divide1 : Product  Inputs=*/
  Gain : Gain  Gain=1/C
  Integrator : Integrator  InitialCondition=E0  LowerSaturationLimit=10
  Product : Product  RndMeth=Zero
  Product1 : Product  RndMeth=Zero
  Saturation : Saturate  UpperLimit=inf  LowerLimit=1e-3
  Sum : Sum  Inputs=|+-
  E : Outport
  iDCm : Outport  Port=2
  wires:
  Divide1/1 -> Sum/1
  Add1/1 -> Divide1/1
  vlabc/1 -> Product1/2
  Demux1/1 -> Add1/1
  Demux1/2 -> Add1/2
  Product1/1 -> Demux1/1
  ilabc/1 -> Product1/1
  Demux1/3 -> Add1/3
  Integrator/1 -> E/1, Saturation/1
  Saturation/1 -> Divide1/2, Divide/2
  Divide/1 -> Sum/2, iDCm/1
  Add/1 -> Divide/1
  isabc/1 -> Product/2
  vsabc/1 -> Product/1
  Gain/1 -> Integrator/1
  Sum/1 -> Gain/1
  Demux/3 -> Add/3
  Demux/2 -> Add/2
  Demux/1 -> Add/1
  Product/1 -> Demux/1

== system Non_WindFarm/FOM/Wind Farm/Wind Turbine Strings/String6/WT5/WFG/Control Electric Generador ==
  note: voltage source converter
  note: Vs_qd_hat(control output)
  note: 10.14
  note: Vs_qd
  note: 4.25
  note: continuous PI
  note: 4.22
  note: 4.22
  parell_ma : Inport
  Q_sa : Inport  Port=2
  isabc : Inport  Port=3
  omega_m : Inport  Port=4
  theta_m : Inport  Port=5
  Constant1 : Constant  Value=0
  Constant2 : Constant  Value=0
  Constant5 : Constant  Value=0
  Divide : Product  Inputs=*/
  Gain : Gain  Gain=-Lq
  Gain1 : Gain  Gain=Ld
  Gain2 : Gain  Gain=lambda_m
  Gain3 : Gain  Gain=P
  Gain4 : Gain  Gain=2/(3*P)
  Gain5 : Gain  Gain=1/lambda_m
  Gain6 : Gain  Gain=2/3
  Gain7 : Gain  Gain=P
  Gain8 : Gain  Gain=1/lambda_m
  Matrix Concatenate : Concatenate  Mode=Multidimensional array  ConcatenateDimension=2
  Memory : Memory  Commented=through
  Mux{,1..3} (4 alike) : Mux  Inputs=2
  PI : Subsystem
  Park : Subsystem
  Product1 : Product  Multiplication=Matrix(*)  RndMeth=Zero
  Product2 : Product  Multiplication=Matrix(*)  RndMeth=Zero
  Product4 : Product  Multiplication=Matrix(*)  RndMeth=Zero
  Sat inf : Subsystem
  Sum : Sum  Inputs=|++
  Sum1 : Sum  Inputs=|+-
  Sum2 : Sum  Inputs=++|
  vscabc : Outport
  wires:
  Gain7/1 -> Park/1(theta_r)
  Park/1(Tthetar) -> Product4/1
  Constant2/1 -> Mux/1
  Gain1/1 -> Mux/2
  Gain/1 -> Mux1/1
  Constant1/1 -> Mux1/2
  Mux/1 -> Matrix Concatenate/1
  Mux1/1 -> Matrix Concatenate/2
  Matrix Concatenate/1 -> Product1/1
  Product4/1 -> Product1/2, Sum1/2
  omega_m/1 -> Gain3/1
  Product1/1 -> Sum/2
  Sum2/1 -> Product2/2
  Sum1/1 -> PI/1(e)
  PI/1(u) -> Sum2/2
  Mux2/1 -> Sum1/1
  theta_m/1 -> Gain7/1
  isabc/1 -> Product4/2
  Product2/1 -> Memory/1
  Gain3/1 -> Gain1/1, Gain2/1, Gain/1, Sat inf/1(in)
  Mux3/1 -> Sum/1
  Gain2/1 -> Mux3/1
  Constant5/1 -> Mux3/2
  Park/2(nTthetar) -> Product2/1
  Sum/1 -> Sum2/1
  Gain4/1 -> Mux2/1
  Gain5/1 -> Gain4/1
  Gain8/1 -> Gain6/1
  Q_sa/1 -> Divide/1
  Memory/1 -> vscabc/1
  parell_ma/1 -> Gain5/1
  Sat inf/1(out) -> Divide/2
  Divide/1 -> Gain8/1
  Gain6/1 -> Mux2/2

== system Non_WindFarm/FOM/Wind Farm/Wind Turbine Strings/String6/WT5/WFG/Control Electric Tensio ==
  note: 6.12
  note: i_control
  note: Kp Ki, + or - ?
  note: 6.15-6.18
  E : Inport
  IDCm : Inport  Port=2
  E* : Constant  Value=Easterisc
  Sum : Sum  Inputs=|++
  Sum1 : Sum  Inputs=|+-
  Transfer Fcn : TransferFcn  Numerator=[Kp Ki]  Denominator=[1 0]
  iDCla : Outport
  wires:
  IDCm/1 -> Sum/2
  Sum1/1 -> Transfer Fcn/1
  E/1 -> Sum1/2
  Sum/1 -> iDCla/1
  Transfer Fcn/1 -> Sum/1
  E*/1 -> Sum1/1

== system Non_WindFarm/FOM/Wind Farm/Wind Turbine Strings/String6/WT5/WFG/Control Mecanic ==
  note: Eq 2.19 ???
  note: ??? theta_a?
  note: Generator nominal speed Wmn
  omega_m : Inport
  Constant : Constant  Value=omegamn
  Gain : Gain  Gain=-KCP
  Math Function : Math  Operator=square  SignedPower=on
  Saturation : Saturate  UpperLimit=inf  LowerLimit=0
  Saturation1 : Saturate  UpperLimit=90  LowerLimit=0
  Subtract : Sum  Inputs=+-
  Transfer Fcn : TransferFcn  Numerator=[Kp Ki]  Denominator=[1 0]
  parell_ma : Outport
  theta_a : Outport  Port=2
  wires:
  omega_m/1 -> Subtract/1, Math Function/1
  Math Function/1 -> Gain/1
  Gain/1 -> parell_ma/1
  Saturation1/1 -> theta_a/1
  Constant/1 -> Subtract/2
  Subtract/1 -> Saturation/1
  Saturation/1 -> Transfer Fcn/1
  Transfer Fcn/1 -> Saturation1/1

== system Non_WindFarm/FOM/Wind Farm/Wind Turbine Strings/String6/WT5/WFG/Control de Corrent de Xarxa2 ==
  vzabc : Inport
  ilabc : Inport  Port=2
  iDCla : Inport  Port=3
  E : Inport  Port=4
  Constant1 : Constant  Value=2*pi*50
  Constant2 : Constant  Value=0
  Constant3 : Constant  Value=[2,-1,-1;0,-sqrt(3),sqrt(3)]
  Constant5 : Constant  Value=2*pi*50
  Constant6 : Constant  Value=[0;0]
  Demux : Demux  Outputs=2
  Demux1 : Demux  Outputs=2
  Divide : Product  Inputs=*/
  Gain1 : Gain  Gain=2/3
  Gain12 : Gain
  Gain2 : Gain  Gain=Ll
  Gain4 : Gain  Gain=Ll
  Gain6 : Gain  Gain=1/3
  Integrator : Integrator
  Memory : Memory  Commented=through
  Mux : Mux  Inputs=2
  Mux1 : Mux  Inputs=2
  PI_d : Subsystem
  Product : Product  RndMeth=Zero
  Product{1..2,11..13} (5 alike) : Product  Multiplication=Matrix(*)  RndMeth=Zero
  Product10 : Product  RndMeth=Zero
  Product3 : Product  RndMeth=Zero
  Scope : Scope
  Selector : Selector  InputPortWidth=2  IndexOptions=Index vector (dialog)  Indices=[1]  OutputSizes=1
  Selector2 : Selector  InputPortWidth=2  IndexOptions=Index vector (dialog)  Indices=[2]  OutputSizes=1
  Step : Step  Time=1e-3  Before=1  After=0  SampleTime=0
  Sum1 : Sum  Inputs=-+|
  Sum2 : Sum  Inputs=+--
  Sum3 : Sum  Inputs=+-
  Sum9 : Sum  Inputs=++|
  Switch : Switch  Criteria=u2 > Threshold  SaturateOnIntegerOverflow=off  InputSameDT=off
  Transfer Fcn : TransferFcn  Numerator=-[1 0.129]  Denominator=[1 0]
  rotacio1 : Subsystem
  vlabc : Outport
  wires:
  Integrator/1 -> rotacio1/1(theta)
  E/1 -> Product10/1
  iDCla/1 -> Product10/2
  PI_d/1(u) -> Demux/1
  Demux/1 -> Sum2/3
  Demux/2 -> Sum3/2
  Sum3/1 -> Mux1/2
  Sum2/1 -> Mux1/1
  Product/1 -> Gain2/1
  Product3/1 -> Gain4/1
  Demux1/2 -> Product3/2
  Demux1/1 -> Product/2
  Gain1/1 -> Mux/1
  Gain4/1 -> Sum2/2
  Gain2/1 -> Sum3/1
  Constant2/1 -> Mux/2
  Memory/1 -> vlabc/1
  Constant1/1 -> Product/1, Product3/1
  Product11/1 -> Product1/2
  Product1/1 -> Scope/1, Selector/1, Selector2/1
  Mux/1 -> Sum1/2
  Product13/1 -> Demux1/1, Sum1/1
  Selector/1 -> Divide/2, Sum2/1
  Mux1/1 -> Product2/2
  rotacio1/2(nT) -> Product2/1
  Divide/1 -> Gain1/1
  Product10/1 -> Divide/1
  Product2/1 -> Memory/1
  Switch/1 -> PI_d/1(e)
  Sum1/1 -> Switch/3
  Constant6/1 -> Switch/1
  Step/1 -> Gain12/1
  Gain12/1 -> Switch/2
  Sum9/1 -> Integrator/1
  Selector2/1 -> Transfer Fcn/1
  Constant5/1 -> Sum9/1
  Transfer Fcn/1 -> Sum9/2
  Constant3/1 -> Gain6/1
  Gain6/1 -> Product12/1, Product11/1
  vzabc/1 -> Product11/2
  ilabc/1 -> Product12/2
  Product12/1 -> Product13/2
  rotacio1/1(T) -> Product13/1, Product1/1

== system Non_WindFarm/FOM/Wind Farm/Wind Turbine Strings/String6/WT5/WFG/Filtre de Xarxa1 ==
  note: Vnl and Vnz? Eq 5.11
  vzabc : Inport
  vlabc : Inport  Port=2
  Gain2 : Gain  Gain=rl
  Gain3 : Gain  Gain=1/Ll
  Integrator : Integrator  InitialCondition=[0;0;0]
  Sum : Sum  Inputs=|+-
  Sum1 : Sum  Inputs=|+-
  ilabc : Outport
  wires:
  vlabc/1 -> Sum/2
  vzabc/1 -> Sum/1
  Gain3/1 -> Integrator/1
  Integrator/1 -> ilabc/1, Gain2/1
  Sum1/1 -> Gain3/1
  Gain2/1 -> Sum1/2
  Sum/1 -> Sum1/1

== system Non_WindFarm/FOM/Wind Farm/Wind Turbine Strings/String6/WT5/WFG/Maquina Sincrona ==
  note: Eq 4.22
  note: park transformation & Inverse
  note: theta_r
  note: Electrical angle=Mechnical angle *Pole Pairs
  note: Omega_r=Omega_m*P
  vsabc : Inport
  omega_m : Inport  Port=2
  theta_m : Inport  Port=3  PortDimensions=1
  Add : Sum  Inputs=+++
  Constant : Constant  Value=-rs/Lq
  Constant1 : Constant  Value=-rs/Ld
  Constant2 : Constant  Value=[1/Lq;0]
  Constant3 : Constant  Value=[1/Lq,0;0,1/Ld]
  Demux : Demux  Outputs=2
  Gain : Gain  Gain=-Ld/Lq
  Gain1 : Gain  Gain=Lq/Ld
  Gain2 : Gain  Gain=-lambda_m
  Gain3 : Gain  Gain=lambda_m
  Gain4 : Gain  Gain=Ld-Lq
  Gain5 : Gain  Gain=3/2*P
  Gain6 : Gain  Gain=P
  Gain7 : Gain  Gain=P
  Integrator : Integrator  InitialCondition=isqd0
  Matrix Concatenate : Concatenate  Mode=Multidimensional array  ConcatenateDimension=2
  Mux : Mux  Inputs=2
  Mux1 : Mux  Inputs=2
  Park : Subsystem
  Product{,2,4..5} (4 alike) : Product  Multiplication=Matrix(*)  RndMeth=Zero
  Product1 : Product  RndMeth=Zero
  Product3 : Product  RndMeth=Zero
  Sum : Sum  Inputs=|++
  isabc : Outport
  parell_m : Outport  Port=2
  wires:
  Constant/1 -> Mux/1
  Gain1/1 -> Mux/2
  Gain/1 -> Mux1/1
  Constant1/1 -> Mux1/2
  omega_m/1 -> Gain6/1
  Mux/1 -> Matrix Concatenate/1
  Mux1/1 -> Matrix Concatenate/2
  Matrix Concatenate/1 -> Product/1
  Product/1 -> Add/1
  Add/1 -> Integrator/1  "disqd"
  Integrator/1 -> Demux/1, Product5/2, Product/2  "isqd"
  Gain2/1 -> Product1/2
  Constant2/1 -> Product1/1
  Product1/1 -> Add/2
  Constant3/1 -> Product2/1
  Product2/1 -> Add/3
  Demux/1 -> Gain3/1, Product3/2
  Product3/1 -> Gain4/1
  Demux/2 -> Product3/1
  Gain3/1 -> Sum/1
  Gain4/1 -> Sum/2
  Sum/1 -> Gain5/1
  Gain5/1 -> parell_m/1
  Gain6/1 -> Gain1/1, Gain/1, Gain2/1
  theta_m/1 -> Gain7/1
  Product4/1 -> Product2/2
  Park/1(Tthetar) -> Product4/1
  Gain7/1 -> Park/1(theta_r)
  Park/2(nTthetar) -> Product5/1
  Product5/1 -> isabc/1
  vsabc/1 -> Product4/2

== system Non_WindFarm/FOM/Wind Farm/Wind Turbine Strings/String6/WT5/WFG/Mecanica nolineal i vent ==
  note: gearbox ration
  note: Gamma_t
  parell_m : Inport
  theta_a : Inport  Port=2
  vw : Inport  Port=3
  Gain1 : Gain  Gain=1/It
  Gain2 : Gain  Gain=nu
  Gain4 : Gain  Gain=nu
  Gain5 : Gain  Gain=nu
  Integrator : Integrator  InitialCondition=omegat0
  Integrator1 : Integrator
  Saturation : Saturate  UpperLimit=inf  LowerLimit=1e-6
  Sum : Sum  Inputs=++|
  Transfer Fcn : TransferFcn  Denominator=[taupitch 1]
  Turbina : Subsystem  mask{rho=1.225, R=R, cs=[0.5 116 0.4 0 0 5 21 0.08 0.035]}
      mask prompts: rho "Densitat de l'aire (Kg/m^3)"; R "Radi (R)"; cs "Constants [c1 c2 .. c9]"
      mask init:
      | A=pi*R^2;
      | c1=cs(1);
      | c2=cs(2);
      | c3=cs(3);
      | c4=cs(4);
      | c5=cs(5);
      | c6=cs(6);
      | c7=cs(7);
      | c8=cs(8);
      | c9=cs(9);
  omega_m : Outport
  theta_m : Outport  Port=2
  Cp : Outport  Port=3
  theta_aleps : Outport  Port=4
  wires:
  Sum/1 -> Gain1/1
  Gain1/1 -> Integrator/1
  Integrator/1 -> Integrator1/1, Gain4/1, Saturation/1
  Turbina/1(parell_turbina) -> Sum/2
  Gain2/1 -> Sum/1
  parell_m/1 -> Gain2/1
  Integrator1/1 -> Gain5/1
  Gain4/1 -> omega_m/1
  Gain5/1 -> theta_m/1
  Saturation/1 -> Turbina/2(omega_aleps)
  Turbina/2(Cp) -> Cp/1
  Transfer Fcn/1 -> theta_aleps/1, Turbina/3(theta_aleps)  "theta_aleps"
  theta_a/1 -> Transfer Fcn/1
  vw/1 -> Turbina/1(velocitat_vent)

== system Non_WindFarm/FOM/Wind Farm/Wind Turbine Strings/String6/WT5/WFG/Park ==
  theta_r : Inport
  Constant4 : Constant  Value=2*pi/3
  Gain7 : Gain  Gain=2/3
  Matrix Concatenate1 : Concatenate  NumInputs=3  Mode=Multidimensional array  ConcatenateDimension=2
  Matrix Concatenate2 : Concatenate  Mode=Multidimensional array  ConcatenateDimension=2
  Mux2 : Mux  Inputs=2
  Mux3 : Mux  Inputs=2
  Mux4 : Mux  Inputs=2
  Mux5 : Mux  Inputs=3
  Mux6 : Mux  Inputs=3
  Sum1 : Sum  Inputs=|++
  Sum2 : Sum  Inputs=|+-
  Trigonometric Function : Trigonometry  Operator=cos
  Trigonometric Function1 : Trigonometry
  Trigonometric Function2 : Trigonometry  Operator=cos
  Trigonometric Function3 : Trigonometry
  Trigonometric Function4 : Trigonometry  Operator=cos
  Trigonometric Function5 : Trigonometry
  Tthetar : Outport
  nTthetar : Outport  Port=2
  wires:
  theta_r/1 -> Sum1/1, Sum2/1, Trigonometric Function/1, Trigonometric Function1/1
  Sum2/1 -> Trigonometric Function2/1, Trigonometric Function3/1
  Sum1/1 -> Trigonometric Function4/1, Trigonometric Function5/1
  Constant4/1 -> Sum2/2, Sum1/2
  Trigonometric Function/1 -> Mux2/1, Mux5/1
  Trigonometric Function1/1 -> Mux2/2, Mux6/1
  Trigonometric Function2/1 -> Mux3/1, Mux5/2
  Trigonometric Function3/1 -> Mux3/2, Mux6/2
  Trigonometric Function4/1 -> Mux4/1, Mux5/3
  Trigonometric Function5/1 -> Mux4/2, Mux6/3
  Mux2/1 -> Matrix Concatenate1/1
  Mux3/1 -> Matrix Concatenate1/2
  Mux4/1 -> Matrix Concatenate1/3
  Matrix Concatenate1/1 -> Gain7/1
  Mux5/1 -> Matrix Concatenate2/1
  Mux6/1 -> Matrix Concatenate2/2
  Gain7/1 -> Tthetar/1
  Matrix Concatenate2/1 -> nTthetar/1

== system Non_WindFarm/FOM/Wind Farm/Wind Turbine Strings/String6/WT6/Transformer-complex/homopolar sequence ==
  note: Vc_filter_qd_bar
  note: Vc_filter_abc_bar
  note: WE
  note: Vc_cable_qd_bar
  note: Vc_cable_abc_bar
  Vc_cable_qd : Inport
  Vc_filter_qd : Inport  Port=2
  Clock : Clock
  Park : Subsystem
  Product{3..5,7} (4 alike) : Product  Multiplication=Matrix(*)  RndMeth=Zero
  homopolar sequence 1 : Subsystem
  homopolar sequence 2 : Subsystem
  we : Gain  Gain=100*pi
  Vc_cable_bar : Outport
  Vc_filter_bar : Outport  Port=2
  wires:
  Product7/1 -> Vc_cable_bar/1
  Product3/1 -> homopolar sequence 1/1(v)
  Vc_filter_qd/1 -> Product3/2
  Vc_cable_qd/1 -> Product4/2
  Product5/1 -> Vc_filter_bar/1
  we/1 -> Park/1(theta_r)
  Clock/1 -> we/1
  homopolar sequence 1/1(v_bar) -> Product5/2
  homopolar sequence 2/1(v_bar) -> Product7/2
  Product4/1 -> homopolar sequence 2/1(v)
  Park/1(Tthetar) -> Product7/1, Product5/1
  Park/2(nTthetar) -> Product4/1, Product3/1

== system Non_WindFarm/FOM/Wind Farm/Wind Turbine Strings/String6/WT6/WFG/Bus Continua1 ==
  note: E=-V_DC?
  note: V_DC/R_DC ?
  note: Eq 5.2-5.5
  ilabc : Inport
  vlabc : Inport  Port=2
  vsabc : Inport  Port=3
  isabc : Inport  Port=4
  Add : Sum  Inputs=+++
  Add1 : Sum  Inputs=+++
  Demux : Demux  Outputs=3
  Demux1 : Demux  Outputs=3
  Divide : Product  Inputs=*/
  Divide1 : Product  Inputs=*/
  Gain : Gain  Gain=1/C
  Integrator : Integrator  InitialCondition=E0  LowerSaturationLimit=10
  Product : Product  RndMeth=Zero
  Product1 : Product  RndMeth=Zero
  Saturation : Saturate  UpperLimit=inf  LowerLimit=1e-3
  Sum : Sum  Inputs=|+-
  E : Outport
  iDCm : Outport  Port=2
  wires:
  Divide1/1 -> Sum/1
  Add1/1 -> Divide1/1
  vlabc/1 -> Product1/2
  Demux1/1 -> Add1/1
  Demux1/2 -> Add1/2
  Product1/1 -> Demux1/1
  ilabc/1 -> Product1/1
  Demux1/3 -> Add1/3
  Integrator/1 -> E/1, Saturation/1
  Saturation/1 -> Divide1/2, Divide/2
  Divide/1 -> Sum/2, iDCm/1
  Add/1 -> Divide/1
  isabc/1 -> Product/2
  vsabc/1 -> Product/1
  Gain/1 -> Integrator/1
  Sum/1 -> Gain/1
  Demux/3 -> Add/3
  Demux/2 -> Add/2
  Demux/1 -> Add/1
  Product/1 -> Demux/1
